simulink model "float_model"  (R2024a)
settings: Solver=VariableStepAuto  StartTime=0.0  StopTime=1  FixedStep=1/(50*16*16)  RelTol=1e-3
undefined symbols (not defined in the file): Radix, SAMPLING_FREQ, signal_1
libraries: dspstat3 x3, dspxfrm3 x1, dspsrcs4 x1, simulink x1
settings Model: SimulationMode=accelerator  Creator=Jan Rosa  LastModifiedBy=Jan Rosa
settings DebuggingCC: SignalRangeChecking=warning

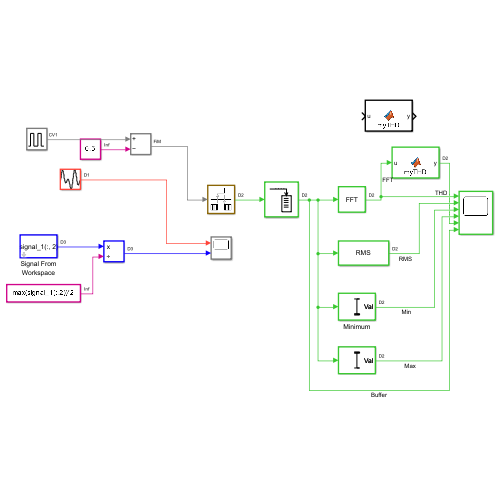
[thumbnail: Simulink's stored preview of the top-level diagram]
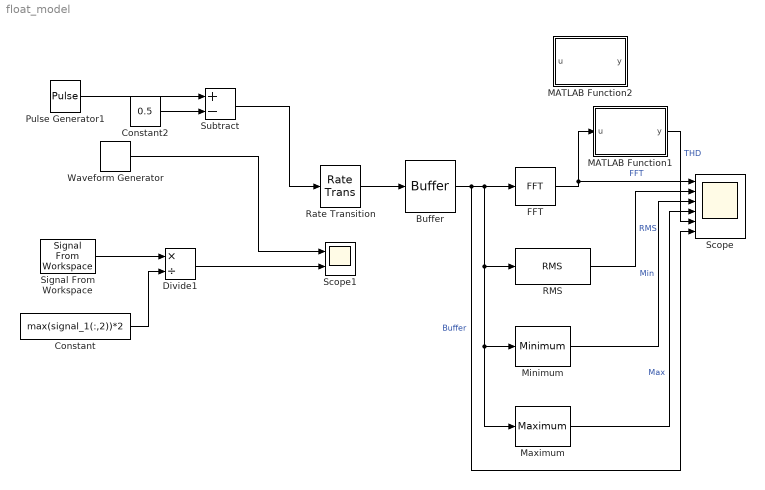
== system float_model ==
  Buffer : Buffer  N=2048  V=2047  OutputFrames=off
  Constant : Constant  Value=max(signal_1(:,2))*2
  Constant2 : Constant  Value=0.5
  Divide1 : Product  Inputs=*/
  FFT : dspxfrm3/FFT  FFTImplementation=Radix-2  CompMethod=Table lookup  TableOpt=NEW  TableOptActive=Speed  BitRevOrder=off  Normalize=on  InheritFFTLength=on  FFTLength=64  WrapInput=on  roundingMode=Ceiling  overflowMode=off  firstCoeffDataTypeStr=Inherit: Same word length as input  firstCoeffLastDataTypeStr=Inherit: Same word length as input  outputMin=[]  outputMax=[]
  MATLAB Function1 : MATLAB Function  TreatAsAtomicUnit=on
  MATLAB Function2 : MATLAB Function  TreatAsAtomicUnit=on
  Maximum : dspstat3/Maximum  operation=maximum  fcn=Value  indexBase=One  operateOver=Each column  Dimension=1  InputProcessing=Columns as channels (frame based)  reset=None  roiEnable=off  roiType=Rectangles  roiPortion=Entire ROI  roiOutput=Individual statistics for each ROI  roiFlag=off  roundingMode=Floor  overflowMode=off  accumDataTypeStr=Inherit: Same as product output  accumLastDataTypeStr=Inherit: Same as product output
  Minimum : dspstat3/Minimum  operation=minimum  fcn=Value  indexBase=One  operateOver=Entire input  Dimension=1  InputProcessing=Columns as channels (frame based)  reset=None  roiEnable=off  roiType=Rectangles  roiPortion=Entire ROI  roiOutput=Individual statistics for each ROI  roiFlag=off  roundingMode=Floor  overflowMode=off
      settings: LibrarySourceBlock=dsphdlsupportstat/Minimum
  Pulse Generator1 : DiscretePulseGenerator  PulseType=Time based  Amplitude=0.999  Period=1/50  PulseWidth=50
  RMS : dspstat3/RMS  run=off  directionMode=Entire input  dimension=1  InputProcessing=Columns as channels (frame based)  reset_popup=None
  Rate Transition : RateTransition  Deterministic=off  OutPortSampleTime=1/SAMPLING_FREQ
  Scope : Scope  NumInputPorts=6
  Scope1 : Scope  NumInputPorts=2
  Signal From Workspace : dspsrcs4/Signal From Workspace  X=signal_1(:, 2)  Ts=signal_1(2, 1)  nsamps=1  OutputAfterFinalValue=Cyclic repetition  ignoreOrWarnInputAndFrameLengths=off  OutputFrames=off
  Subtract : Sum  Inputs=+-
  Waveform Generator : simulink/Sources/Waveform Generator  OutMin=[]  OutMax=[]  OutDataTypeStr=double  SelectedSignal=1  Signals=0.99*sin(0.5, 50*2*pi, 0)  BlockNames=MultiportSwitch_ec0194048af0448  SampleTime=1/(SAMPLING_FREQ*2)
  wires:
  Buffer/1 -> Scope/6, FFT/1, Maximum/1, Minimum/1, RMS/1  "Buffer"
  Divide1/1 -> Scope1/2
  RMS/1 -> Scope/2  "RMS"
  Minimum/1 -> Scope/3  "Min"
  Maximum/1 -> Scope/4  "Max"
  Rate Transition/1 -> Buffer/1
  FFT/1 -> MATLAB Function1/1(u), Scope/1  "FFT"
  Signal From Workspace/1 -> Divide1/1
  Constant/1 -> Divide1/2
  MATLAB Function1/1(y) -> Scope/5  "THD"
  Waveform Generator/1 -> Scope1/1
  Constant2/1 -> Subtract/2
  Pulse Generator1/1 -> Subtract/1
  Subtract/1 -> Rate Transition/1

== matlab function float_model/MATLAB Function2 ==
  data: u input; y output
function y = myTHD(u)

    main_frequency_index = 9;
    u_abs = abs(u);
    halfway_index = floor(length(u_abs) / 2); % Calculate the halfway point
    u_abs_square = u_abs(main_frequency_index+1:halfway_index).^2;
    u_abs_SM = sum(u_abs_square);
    
y = (sqrt(u_abs_SM))/u_abs(main_frequency_index);

== matlab function float_model/MATLAB Function1 ==
  data: u input; y output
function y = myTHD(u)

    main_frequency_index = 9;
    u_abs = abs(u);
    halfway_index = floor(length(u_abs) / 2); % Calculate the halfway point
    u_abs_square = u_abs(main_frequency_index+1:halfway_index).^2;
    u_abs_SM = sum(u_abs_square);
    
y = (sqrt(u_abs_SM))/u_abs(main_frequency_index);
